simulink model "BMS_Harness_StateMachine_1"  (R2024a)
settings: configuration reference "AutosarConfig" (kept outside this file)
libraries: SignalEditorBlockLib x1
settings Model: DataDictionary=BMS_Software_DD.sldd  Creator=smuckati  LastModifiedBy=smuckati
settings ConfigSetRef: SourceName=AutosarConfig

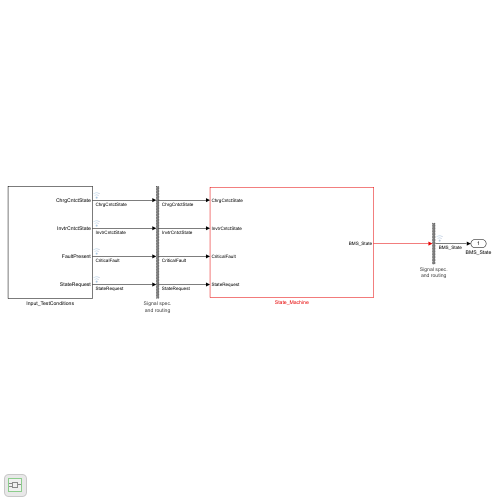
[thumbnail: Simulink's stored preview of the top-level diagram]
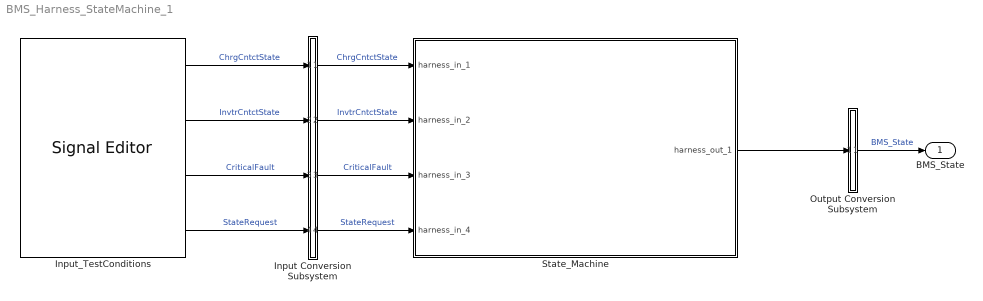
== system BMS_Harness_StateMachine_1 ==
  Input Conversion Subsystem : Subsystem  Tag=__SLT_ICS__  Description=|
      | Signal spec.
      | and routing
      settings: AttributesFormatString=%<Description>
  Input_TestConditions : SignalEditorBlockLib/Signal Editor  FileName=State_Machine_HarnessInputs.mat  ActiveScenario=Standby  ActiveSignal=InvtrCntctState  IsBus=off  OutputBusObjectStr=Bus: BusObject  SampleTime=0.1  Interpolate=off  ZeroCross=off  OutputAfterFinalValue=Setting to zero  Unit=inherit  PreserveSignalName=on  ApplySigPropsToAllScenarios=off  ApplySigPropsToAllSignals=off
  Output Conversion Subsystem : Subsystem  Tag=__SLT_OCS__  Description=|
      | Signal spec.
      | and routing
      settings: AttributesFormatString=%<Description>
  State_Machine : Subsystem  Tag=__SL_testing_harness_stub_
  BMS_State : Outport
  wires:
  Input_TestConditions/1 -> Input Conversion Subsystem/1(Inport_1)  "ChrgCntctState"
  Input_TestConditions/2 -> Input Conversion Subsystem/2(Inport_2)  "InvtrCntctState"
  Input_TestConditions/3 -> Input Conversion Subsystem/3(Inport_3)  "CriticalFault"
  Input_TestConditions/4 -> Input Conversion Subsystem/4(Inport_4)  "StateRequest"
  Output Conversion Subsystem/1(Outport_1) -> BMS_State/1  "BMS_State"
  Input Conversion Subsystem/1(Outport_1) -> State_Machine/1(harness_in_1)  "ChrgCntctState"
  Input Conversion Subsystem/2(Outport_2) -> State_Machine/2(harness_in_2)  "InvtrCntctState"
  Input Conversion Subsystem/3(Outport_3) -> State_Machine/3(harness_in_3)  "CriticalFault"
  Input Conversion Subsystem/4(Outport_4) -> State_Machine/4(harness_in_4)  "StateRequest"
  State_Machine/1(harness_out_1) -> Output Conversion Subsystem/1(Inport_1)

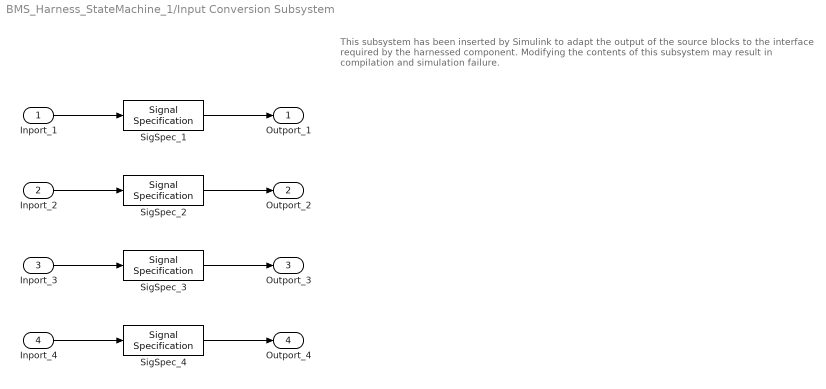
== system BMS_Harness_StateMachine_1/Input Conversion Subsystem ==
  note: This subsystem has been inserted by Simulink to adapt the output of the source blocks to the interface required by the harnessed component.
      |  Modifying the contents of this subsystem may result in compilation and simulation failure.
  Inport_1 : Inport
  Inport_2 : Inport  Port=2
  Inport_3 : Inport  Port=3
  Inport_4 : Inport  Port=4
  SigSpec_1 : SignalSpecification  OutDataTypeStr=Enum: Contact  Dimensions=[1]  SampleTime=0.1
  SigSpec_2 : SignalSpecification  OutDataTypeStr=Enum: Contact  Dimensions=[1]  SampleTime=0.1
  SigSpec_3 : SignalSpecification  OutDataTypeStr=boolean  Dimensions=[1]  SampleTime=0.1
  SigSpec_4 : SignalSpecification  OutDataTypeStr=Enum: SRE  Dimensions=[1]  SampleTime=0.1
  Outport_1 : Outport
  Outport_2 : Outport  Port=2
  Outport_3 : Outport  Port=3
  Outport_4 : Outport  Port=4
  wires:
  SigSpec_1/1 -> Outport_1/1
  Inport_1/1 -> SigSpec_1/1
  SigSpec_2/1 -> Outport_2/1
  Inport_2/1 -> SigSpec_2/1
  SigSpec_3/1 -> Outport_3/1
  Inport_3/1 -> SigSpec_3/1
  SigSpec_4/1 -> Outport_4/1
  Inport_4/1 -> SigSpec_4/1

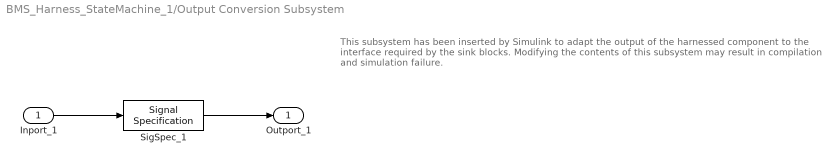
== system BMS_Harness_StateMachine_1/Output Conversion Subsystem ==
  note: This subsystem has been inserted by Simulink to adapt the output of the harnessed component to the interface required by the sink blocks.
      |  Modifying the contents of this subsystem may result in compilation and simulation failure.
  Inport_1 : Inport
  SigSpec_1 : SignalSpecification  OutDataTypeStr=Enum: BMS_State_Enum  Dimensions=[1]  SampleTime=0.1
  Outport_1 : Outport
  wires:
  Inport_1/1 -> SigSpec_1/1
  SigSpec_1/1 -> Outport_1/1

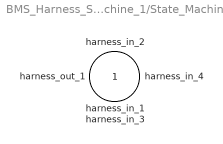
== system BMS_Harness_StateMachine_1/State_Machine ==
  harness_in_1 : Inport
  harness_in_2 : Inport  Port=2
  harness_in_3 : Inport  Port=3
  harness_in_4 : Inport  Port=4
  harness_out_1 : Outport
